simulink model "simrfV2_lte_receiver"  (R2022a)
settings: Solver=VariableStepAuto  StartTime=0  StopTime=0.001  RelTol=1e-3
InitFcn:
  | % Default workspace values
  | 
  | if ~exist('SNRdB')
  |      SNRdB = 57;
  | end
  | 
  | if ~exist('SymbolPower')
  |      SymbolPower = 1.5514e-10;
  | end
  | 
  | if ~exist('txWaveform')
  |      txWaveform = timeseries(complex(0,0),0);
  | end
  | 
  | if ~exist('SamplePeriod')
  |      SamplePeriod = 1/7680000;
  | end
  | 
  | if ~exist('h')
  |      h = 1;
  | end
  | 
  | if ~exist('Es')
  |      Es = 7.9433e-8;
  | end
values from neighbouring files (symbols this model uses):
  N = 3    [RFReceiverModelingForLteReceptionExample.m]
undefined symbols (not defined in the file or in its folder): magnitude, physconst, S
libraries: simrfV2util1 x4, simrfV2elements x3, simulink_extras x2, dspstat3 x2, dspmathops x2, commrflib2 x1, simrfV2systems x1, simrfV2sources1 x1
settings Model: SimulationMode=accelerator  Creator=The MathWorks, Inc.  LastModifiedBy=The MathWorks, Inc.
settings SolverCC: ExtrapolationOrder=1  AlgebraicLoopSolver=TrustRegion  MaxZcPerStep=1
settings DataIOCC: ExternalInput=txWaveform  SaveFinalState=on  SaveOperatingPoint=on  SaveOutput=off  SignalLogging=off  DSMLogging=off  SaveTime=off  ReturnWorkspaceOutputs=off  OutputSaveName=rx
settings OptimizationCC: EfficientMapNaN2IntZero=off  LifeSpan=inf
settings DebuggingCC: UnderspecifiedInitializationDetection=Classic  MergeDetectMultiDrivingBlocksExec=none  SolverPrmCheckMsg=warning  UnconnectedInputMsg=warning  UnconnectedOutputMsg=warning  UnconnectedLineMsg=warning  AllowSymbolicDim=off  SFUnexpectedBacktrackingDiag=warning  SFNoUnconditionalDefaultTransitionDiag=warning  SFExecutionAtInitializationDiag=none  SFMachineParentedDataDiag=warning  ArithmeticOperatorsInVariantConditions=warning
settings HardwareCC: ProdBitPerPointer=32  ProdBitPerSizeT=32  ProdBitPerPtrDiffT=32  ProdLargestAtomicFloat=None  ProdIntDivRoundTo=Undefined  ProdEndianess=Unspecified  ProdWordSize=32  ProdHWDeviceType=32-bit Generic  TargetBitPerLong=64  TargetBitPerPointer=64  TargetBitPerSizeT=64  TargetBitPerPtrDiffT=64  TargetLongLongMode=on  TargetIntDivRoundTo=Zero  TargetEndianess=LittleEndian  TargetWordSize=64  TargetHWDeviceType=MATLAB Host  ProdEqTarget=off
settings ModelReferenceCC: PropagateSignalLabelsOutOfModel=off
settings SFSimCC: SimUseLocalCustomCode=off  CustomCodeUndefinedFunction=UseInterfaceOnly
settings RTWCC: RTWUseLocalCustomCode=off  DLArmComputeVersion=19.05
settings CodeAppCC: MaxIdLength=128  StateflowObjectComments=on
settings GRTTargetCC: TargetLangStandard=C89/C90 (ANSI)  CombineOutputUpdateFcns=off  GRTInterface=on
settings ConfigComp: CovMetricSettings=dw  CovSaveCumulativeToWorkspaceVar=on  CovSaveSingleToWorkspaceVar=on  CovExternalEMLEnable=off  CovSFcnEnable=off
settings SimscapeCC: SimscapeNormalizeSystem=off  SimscapeNominalValues="[{\"value\":\"10\",\"unit\":\"V\"},{\"value\":\"1\",\"unit\":\"A\"},{\"value\":\"10\",\"unit\":\"N*m\"},{\"value\":\"10\",\"unit\":\"bar\"},{\"value\":\"100\",\"unit\":\"kJ/kg\"},{\"value\":\"1\",\"unit\":\"kW\"},{\"value\":\"300\",\"unit\":\"K\"},{\"value\":\"100\",\"unit\":\"cm^3/s\"},{\"value\":\"1\",\"unit\":\"kN\"},{\"value\":\"1\",\"unit\":\"g/cm^3\"},{\"value\":\"1\",\"unit\":\"l\"},{\"value\":\"1\",\"unit\":\"cm^2\"},{\"value\":\"60\",\"unit\":\"Hz\"}]"

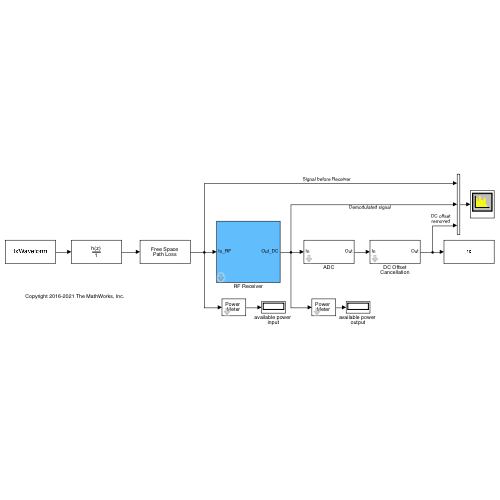
[thumbnail: Simulink's stored preview of the top-level diagram]
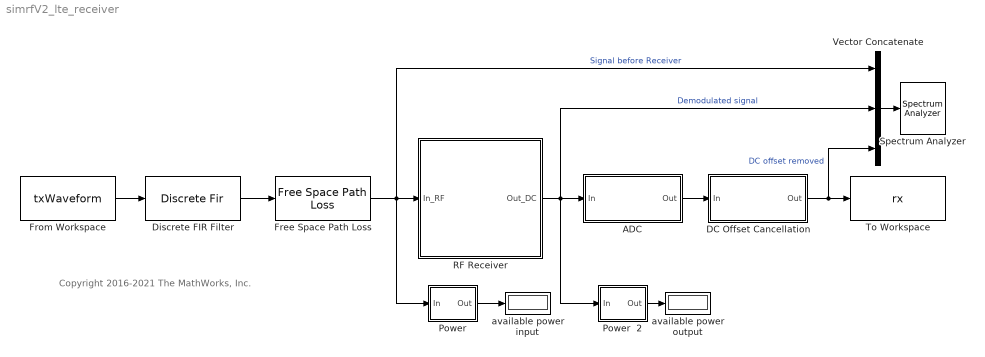
== system simrfV2_lte_receiver ==
  note: Copyright 2016-2021 The MathWorks, Inc.
  ADC : Subsystem  mask{Pmax=-30, N=10}
      mask prompts: Pmax "Full scale power (dBm)"; N "Number of bits"
  DC Offset Cancellation : Subsystem  mask(DC Offset Cancellation){N=32, V=N/2, ic=5e-4*(1+1j)}
      mask prompts: N "Lenght of Averaging Filter (Samples):"; V "Buffer Overlap:"; ic "Initial Condition"
      mask help: Remove the DC offset by averaging the input signal.
      mask init:
      | V = N/2;
      mask Help:
      | Estimate the DC offeset of a signal using a running average filter, and removes it from the signal itself
      | This model uses components from the DSP System Toolbox.
      mask TypeOptions N: Buffer/N
      mask TypeOptions V: Buffer/V
      mask TypeOptions ic: Buffer/ic
  Discrete FIR Filter : DiscreteFir  Coefficients=h  InputProcessing=Columns as channels (frame based)
  Free Space Path Loss : commrflib2/Free Space Path Loss  mode=Decibels  dB=-10*log10(Es)  d=0.100  fc=1920
      settings: SourceProductBaseCode=CM
  From Workspace : FromWorkspace  VariableName=txWaveform  SampleTime=SamplePeriod  Interpolate=off  OutputAfterFinalValue=Setting to zero
  "Power  " : Subsystem  mask{R=1}
      mask prompts: R "Reference Impedance [Ohm]"
      mask DialogControl DescGroupVar Prompt: Power Meter
      mask Display: disp('Power \nMeter')
  Power  2 : Subsystem  mask{R=1}
      mask prompts: R "Reference Impedance [Ohm]"
      mask DialogControl DescGroupVar Prompt: Power Meter
      mask Display: disp('Power \nMeter')
  RF Receiver : Subsystem  mask(LTE RF Direct Conversion Receiver){StepSize=SamplePeriod, CarrierFreq=2.14, S21=11.4, S12=-33, S11=-20, S22=-19, NF_LNA=1.2, IP3_LNA=-6.6, P1dB_LNA=-12, Gain_Demod=2.3, Gain_Mismatch=0.05, Phase_Mismatch=2, Isolation=65, IP2_Demod=56, IP3_Demod=25.9, NF_Demod=10.9, PN_f=[100e3 500e3 1e6], PN_c=[-110 -139 -145], Gain_VGA=15, NF_VGA=8.3, IP3_VGA=11.3, P1dB_VGA=-2.5}
      mask prompts: StepSize "Sample Time (s)"; CarrierFreq "Center Frequency (GHz)"; S21 "Gain (dB)"; S12 "Reverse Isolation (dB)"; S11 "Input Return Loss (dB)"; S22 "Output Return Loss (dB)"; NF_LNA "Noise Figure (dB)"; IP3_LNA "Input Referred IP3 (dBm)"; P1dB_LNA "1dB Compression Point (dBm)"; Gain_Demod "Gain (dB)"; Gain_Mismatch "I/Q Gain Mismatch (dB)"; Phase_Mismatch "I/Q Phase Mismatch (Deg)"; Isolation "RF to LO Isolation (dB)"; IP2_Demod "Input Referred IP2 (dBm)"; IP3_Demod "Input Referred IP3 (dBm)"; NF_Demod "Noise figure (dB)"; PN_f "Phase Noise Frequency Vector (Hz)"; PN_c "PhaseNoise Level (dBc/Hz)"; Gain_VGA "Gain (dB)"; NF_VGA "Noise Figure (dB)"; IP3_VGA "Input Referred IP3 (dBm)"; P1dB_VGA "1dB Compression Point (dBm)"
      mask help: Estimate the impact of non linearity, noise, DC offset, mismatches and imbalance.
      mask init:
      | Sparam_LNA = 10.^([S11 S12; S21 S22]./20);
      mask Help:
      | Estimate the impact of non linearity, noise, DC offset, mismatches and imbalance introduced by an RF chain composed by an LNA, Direct Conversion demodulator and VGA.
      | This model uses components from the RF Blockset Circuit Envelope library.
      mask DialogControl Container4 Prompt: Simulation Parameters
      mask DialogControl Container13 Prompt: LNA
      mask DialogControl Container17 Prompt: I-Q Demodulator
      mask DialogControl Container18 Prompt: VGA
  Spectrum Analyzer : SpectrumAnalyzer
  To Workspace : ToWorkspace  VariableName=rx  SampleTime=SamplePeriod
      settings: Save2DSignal=2-D array (concatenate along first dimension)
  Vector Concatenate : Concatenate  NumInputs=3  Mode=Multidimensional array  ConcatenateDimension=2
  available power input : Display
  available power output : Display
  wires:
  "Power  "/1(Out) -> available power input/1
  Discrete FIR Filter/1 -> Free Space Path Loss/1
  DC Offset Cancellation/1(Out) -> Vector Concatenate/3, To Workspace/1  "DC offset removed"
  From Workspace/1 -> Discrete FIR Filter/1
  Vector Concatenate/1 -> Spectrum Analyzer/1
  ADC/1(Out) -> DC Offset Cancellation/1(In)
  Power  2/1(Out) -> available power output/1
  RF Receiver/1(Out_DC) -> Power  2/1(In), Vector Concatenate/2, ADC/1(In)  "Demodulated signal"
  Free Space Path Loss/1 -> Vector Concatenate/1, "Power  "/1(In), RF Receiver/1(In_RF)  "Signal before Receiver"

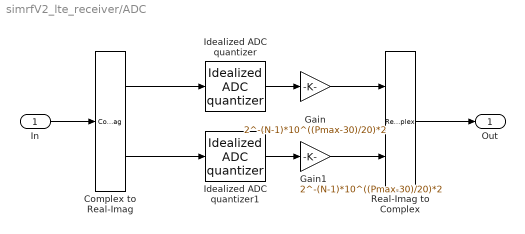
== system simrfV2_lte_receiver/ADC ==
  In : Inport
  Complex to Real-Imag : ComplexToRealImag
  Gain : Gain  Gain=2^-(N-1)*10^((Pmax-30)/20)*2
  Gain1 : Gain  Gain=2^-(N-1)*10^((Pmax-30)/20)*2
  Idealized ADC quantizer : simulink_extras/Additional Discrete/Idealized ADC quantizer  NumberOfConverterBits=N  Vmin=-10^((Pmax-30)/20)*2  Vmax=10^((Pmax-30)/20)*2  OutputDataType=double  OutputNegativeValues=on
  Idealized ADC quantizer1 : simulink_extras/Additional Discrete/Idealized ADC quantizer  NumberOfConverterBits=N  Vmin=-10^((Pmax-30)/20)*2  Vmax=10^((Pmax-30)/20)*2  OutputDataType=double  OutputNegativeValues=on
  Real-Imag to Complex : RealImagToComplex
  Out : Outport  VectorParamsAs1DForOutWhenUnconnected=off
  wires:
  Real-Imag to Complex/1 -> Out/1
  Complex to Real-Imag/1 -> Idealized ADC quantizer/1
  In/1 -> Complex to Real-Imag/1
  Complex to Real-Imag/2 -> Idealized ADC quantizer1/1
  Idealized ADC quantizer/1 -> Gain/1
  Idealized ADC quantizer1/1 -> Gain1/1
  Gain/1 -> Real-Imag to Complex/1
  Gain1/1 -> Real-Imag to Complex/2

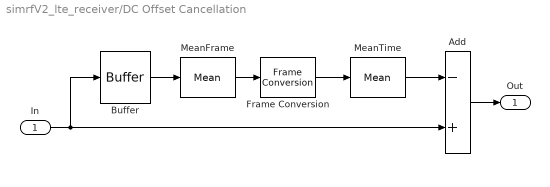
== system simrfV2_lte_receiver/DC Offset Cancellation ==
  In : Inport
  Add : Sum  Inputs=-+
  Buffer : Buffer  N=N  V=V  ic=ic
  Frame Conversion : FrameConversion  OutFrame=Sample-based
  MeanFrame : dspstat3/Mean  run=on  InputProcessing=Columns as channels (frame based)  reset_popup=None  directionMode=Entire input  dimension=1  roiEnable=off  roiType=Rectangles  roiPortion=Entire ROI  roiOutput=Individual statistics for each ROI  roiFlag=off  roundingMode=Floor  overflowMode=off  outputDataTypeStr=Inherit: Same as accumulator  outputMin=[]  outputMax=[]  outputLastDataTypeStr=Inherit: Same as accumulator
  MeanTime : dspstat3/Mean  run=off  InputProcessing=Columns as channels (frame based)  reset_popup=None  directionMode=Entire input  dimension=1  roiEnable=off  roiType=Rectangles  roiPortion=Entire ROI  roiOutput=Individual statistics for each ROI  roiFlag=off  roundingMode=Floor  overflowMode=off  outputDataTypeStr=Inherit: Same as accumulator  outputMin=[]  outputMax=[]  outputLastDataTypeStr=Inherit: Same as accumulator
  Out : Outport  VectorParamsAs1DForOutWhenUnconnected=off
  wires:
  Frame Conversion/1 -> MeanTime/1
  MeanTime/1 -> Add/1
  Add/1 -> Out/1
  MeanFrame/1 -> Frame Conversion/1
  In/1 -> Add/2, Buffer/1
  Buffer/1 -> MeanFrame/1

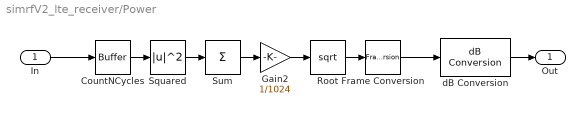
== system simrfV2_lte_receiver/Power   ==
  In : Inport
  CountNCycles : Buffer  N=1024
  Frame Conversion : FrameConversion  OutFrame=Sample-based
  Gain2 : Gain  Gain=1/1024
  Root : Sqrt
  Squared : Math  Operator=magnitude^2  SignedPower=on
  Sum : Sum  Inputs=+
  dB Conversion : dspmathops/dB Conversion  dBtype=dBm  intype=Amplitude  R=R  fuzz=on
  Out : Outport  VectorParamsAs1DForOutWhenUnconnected=off
  wires:
  dB Conversion/1 -> Out/1
  In/1 -> CountNCycles/1
  Frame Conversion/1 -> dB Conversion/1
  CountNCycles/1 -> Squared/1
  Squared/1 -> Sum/1
  Sum/1 -> Gain2/1
  Root/1 -> Frame Conversion/1
  Gain2/1 -> Root/1

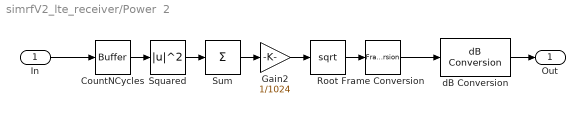
== system simrfV2_lte_receiver/Power  2 ==
  In : Inport
  CountNCycles : Buffer  N=1024
  Frame Conversion : FrameConversion  OutFrame=Sample-based
  Gain2 : Gain  Gain=1/1024
  Root : Sqrt
  Squared : Math  Operator=magnitude^2  SignedPower=on
  Sum : Sum  Inputs=+
  dB Conversion : dspmathops/dB Conversion  dBtype=dBm  intype=Amplitude  R=R  fuzz=on
  Out : Outport  VectorParamsAs1DForOutWhenUnconnected=off
  wires:
  dB Conversion/1 -> Out/1
  In/1 -> CountNCycles/1
  Frame Conversion/1 -> dB Conversion/1
  CountNCycles/1 -> Squared/1
  Squared/1 -> Sum/1
  Sum/1 -> Gain2/1
  Root/1 -> Frame Conversion/1
  Gain2/1 -> Root/1

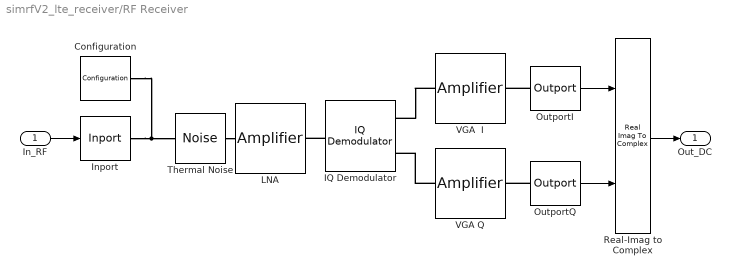
== system simrfV2_lte_receiver/RF Receiver ==
  In_RF : Inport
  Configuration : simrfV2util1/Configuration  AutoFreq=off  Tones=CarrierFreq GHz  Harmonics=3  NormalizeCarrierPower=on  SolverType=Auto  UseCCode=on  StepSize=StepSize s  AddNoise=on  defaultRNG=on  Seed=0  Temperature=290.0 K  SolverDelFlag=0  AbsTol=1e-6  RelTol=1e-3  MaxIter=10  ErrorEstimationType=2-norm over all variables  EnableInterpFilter=off  HiddenFIRfilterControllerParam=off  SmallSignalApprox=off  AllSimFreqs=on  SimFreqs=[] Hz  SimFreqsInternal=[]  SamplesPerFrame=1
      settings: SourceProductBaseCode=RB
  IQ Demodulator : simrfV2systems/IQ Demodulator  classname=iqdemod  Source_linear_gain=Available power gain  linear_gain=Gain_Demod dB  Poly_Coeffs=[0 1]  LOFreq=CarrierFreq GHz  Zin=50  Zout=50  AddIRFilter=off  AddCSFilters=on  InternalGrounding=on  ForceNextInit=off  Source_Poly=Even and odd order  IPType=Input  IP2=IP2_Demod dBm  IP3=IP3_Demod dBm  P1dB=inf dBm  Psat=inf dBm  Gcomp=inf dBm  NF=NF_Demod  GainMismatch=Gain_Mismatch dB  PhaseMismatch=Phase_Mismatch deg  Isolation=Isolation dB  AddPhaseNoise=on  PhaseNoiseOffset=PN_f  PhaseNoiseLevel=PN_c  AutoImpulseLengthPN=on  ImpulseLengthPN=1e-10  ImpulseLength_unitPN=s  DesignMethodIR=Ideal  ResponseTypeIR=Highpass  ImplementationIR=LC Tee  ImplementationIdealIR=Constant per carrier  ImplementationRationalIR=Transfer function  UseFilterOrderIR=on  FilterOrderIR=3  PassFreq_lpIR=1  PassFreq_lp_unitIR=GHz  PassFreq_hpIR=2  PassFreq_hp_unitIR=GHz  PassFreq_bpIR=[2 3]  PassFreq_bp_unitIR=GHz  PassFreq_bsIR=[1 4]  PassFreq_bs_unitIR=GHz  PassAttenIR=10*log10(2)  StopFreq_lpIR=2  StopFreq_lp_unitIR=GHz  StopFreq_hpIR=1  StopFreq_hp_unitIR=GHz  StopFreq_bpIR=[1.5 3.5]  StopFreq_bp_unitIR=GHz  StopFreq_bsIR=[2.1 2.9]  StopFreq_bs_unitIR=GHz  StopAttenIR=40  RsrcIR=50  RloadIR=50  AutoImpulseLengthIR=on  ImpulseLengthIR=1e-10  ImpulseLength_unitIR=s  DesignMethodCS=Ideal  ResponseTypeCS=Lowpass  ImplementationCS=LC Tee  ImplementationIdealCS=Constant per carrier  ImplementationRationalCS=Transfer function  UseFilterOrderCS=on  FilterOrderCS=3  PassFreq_lpCS=1  PassFreq_lp_unitCS=GHz  PassFreq_hpCS=2  PassFreq_hp_unitCS=GHz  PassFreq_bpCS=[2 3]  PassFreq_bp_unitCS=GHz  PassFreq_bsCS=[1 4]  PassFreq_bs_unitCS=GHz  PassAttenCS=10*log10(2)  StopFreq_lpCS=2  StopFreq_lp_unitCS=GHz  StopFreq_hpCS=1  StopFreq_hp_unitCS=GHz  StopFreq_bpCS=[1.5 3.5]  StopFreq_bp_unitCS=GHz  StopFreq_bsCS=[2.1 2.9]  StopFreq_bs_unitCS=GHz  StopAttenCS=40  RsrcCS=50  RloadCS=50  AutoImpulseLengthCS=on  ImpulseLengthCS=1e-10  ImpulseLength_unitCS=s
      settings: SourceProductBaseCode=RB
  Inport : simrfV2util1/Inport  SimulinkInputSignalType=Power  CarrierFreq=CarrierFreq GHz  ZS=50  InternalGrounding=on
      settings: SourceProductBaseCode=RB
  LNA : simrfV2elements/Amplifier  classname=amplifier  DataSource=Network-parameters  File=unitygain.s2p  Paramtype=S-parameters  Sparam=Sparam_LNA  SparamFreq=CarrierFreq GHz  SparamZ0=50  Residues=0  Poles=0  DF={0 0; 1 0}  Source_linear_gain=Data source  linear_gain=18 dB  AmAmAmPmTable=[-25,5,-1;-10,20,-2;0,27,5;5,28,12]  Zin=50  Zout=50  Source_Poly=Odd order  Poly_Coeffs=[0 1]  IPType=Input  IP2=inf dBm  IP3=IP3_LNA dBm  P1dB=P1dB_LNA dBm  Psat=inf dBm  Gcomp=inf dBm  InternalGrounding=on  SourceFreq=Extracted from data source  PlotFreq=1 Hz  PlotType=X-Y plane  YParam1=S(2,1)  YFormat1=Magnitude (decibels)  YParam2=None  YFormat2=Magnitude (decibels)  YOption=Linear  XOption=Linear  SparamRepresentation=Frequency domain  FitTol=-40  FitOpt=Fit individually  MaxPoles=48  AutoImpulseLength=off  ImpulseLength=0 s  MagModeling=off  AddNoise=on  NoiseType=Noise figure  NoiseDist=White  NF=NF_LNA  MinNF=0  Gopt=0  RN=0  CarrierFreq=0 Hz  NoiseAutoImpulseLength=on  NoiseImpulseLength=1e-10 s  ConstS21NL=on  OpFreq=0 Hz  SetOpFreqAsMaxS21=on
      settings: SourceProductBaseCode=RB
  OutportI : simrfV2util1/Outport  SensorType=Power  OutputFormat=Real Passband  CarrierFreq=0 GHz  ZL=50  InternalGrounding=on  StepSize=-1 s  AutoStep=off
      settings: SourceProductBaseCode=RB
  OutportQ : simrfV2util1/Outport  SensorType=Power  OutputFormat=Real Passband  CarrierFreq=0 GHz  ZL=50  InternalGrounding=on  StepSize=-1 s  AutoStep=off
      settings: SourceProductBaseCode=RB
  Real-Imag to Complex : RealImagToComplex
  Thermal Noise : simrfV2sources1/Noise  SimulinkInputSignalType=Ideal voltage  NoiseType=White  NoisePSD=4*physconst('Boltzmann')*290*50  CarrierFreq=0 Hz  AutoImpulseLength=on  ImpulseLength=1e-10 s  InternalGrounding=off
      settings: SourceProductBaseCode=RB
  VGA  I : simrfV2elements/Amplifier  classname=amplifier  DataSource=Data file  File=unitygain.s2p  Paramtype=S-parameters  Sparam=[0 0;1 0]  SparamFreq=1e9 Hz  SparamZ0=50  Residues=0  Poles=0  DF={0 0; 1 0}  Source_linear_gain=Available power gain  linear_gain=Gain_VGA dB  AmAmAmPmTable=[-25,5,-1;-10,20,-2;0,27,5;5,28,12]  Zin=50  Zout=50  Source_Poly=Odd order  Poly_Coeffs=[0 1]  IPType=Input  IP2=19.5 dBm  IP3=IP3_VGA dBm  P1dB=P1dB_VGA dBm  Psat=inf dBm  Gcomp=inf dBm  InternalGrounding=on  SourceFreq=Extracted from data source  PlotFreq=0 Hz  PlotType=X-Y plane  YParam1=S(1,1)  YFormat1=Magnitude (decibels)  YParam2=None  YFormat2=Magnitude (decibels)  YOption=Linear  XOption=Linear  SparamRepresentation=Time domain (rationalfit)  FitTol=-40  FitOpt=Share all poles  MaxPoles=48  AutoImpulseLength=off  ImpulseLength=0 s  MagModeling=off  AddNoise=on  NoiseType=Noise figure  NoiseDist=White  NF=NF_VGA  MinNF=0  Gopt=0  RN=0  CarrierFreq=0 Hz  NoiseAutoImpulseLength=on  NoiseImpulseLength=1e-10 s  ConstS21NL=on  OpFreq=0 Hz  SetOpFreqAsMaxS21=on
      settings: SourceProductBaseCode=RB
  VGA Q : simrfV2elements/Amplifier  classname=amplifier  DataSource=Data file  File=unitygain.s2p  Paramtype=S-parameters  Sparam=[0 0;1 0]  SparamFreq=1e9 Hz  SparamZ0=50  Residues=0  Poles=0  DF={0 0; 1 0}  Source_linear_gain=Available power gain  linear_gain=Gain_VGA dB  AmAmAmPmTable=[-25,5,-1;-10,20,-2;0,27,5;5,28,12]  Zin=50  Zout=50  Source_Poly=Odd order  Poly_Coeffs=[0 1]  IPType=Input  IP2=19.5 dBm  IP3=IP3_VGA dBm  P1dB=P1dB_VGA dBm  Psat=inf dBm  Gcomp=inf dBm  InternalGrounding=on  SourceFreq=Extracted from data source  PlotFreq=0 Hz  PlotType=X-Y plane  YParam1=S(1,1)  YFormat1=Magnitude (decibels)  YParam2=None  YFormat2=Magnitude (decibels)  YOption=Linear  XOption=Linear  SparamRepresentation=Time domain (rationalfit)  FitTol=-40  FitOpt=Share all poles  MaxPoles=48  AutoImpulseLength=off  ImpulseLength=0 s  MagModeling=off  AddNoise=on  NoiseType=Noise figure  NoiseDist=White  NF=NF_VGA  MinNF=0  Gopt=0  RN=0  CarrierFreq=0 Hz  NoiseAutoImpulseLength=on  NoiseImpulseLength=1e-10 s  ConstS21NL=on  OpFreq=0 Hz  SetOpFreqAsMaxS21=on
      settings: SourceProductBaseCode=RB
  Out_DC : Outport  VectorParamsAs1DForOutWhenUnconnected=off
  wires:
  Real-Imag to Complex/1 -> Out_DC/1
  OutportI/1 -> Real-Imag to Complex/1
  OutportQ/1 -> Real-Imag to Complex/2
  In_RF/1 -> Inport/1
  connections:
  OutportI/LConn1 -- VGA  I/RConn1
  VGA  I/LConn1 -- IQ Demodulator/RConn1
  VGA Q/LConn1 -- IQ Demodulator/RConn2
  IQ Demodulator/LConn1 -- LNA/RConn1
  OutportQ/LConn1 -- VGA Q/RConn1
  Thermal Noise/LConn1 -- LNA/LConn1
  Configuration/LConn1 -- Thermal Noise/RConn1 -- Inport/RConn1
